simulink model "periodicSwitchTest"  (Simulink 7.9)
settings: Solver=ode45  StartTime=0.0  StopTime=60  MaxStep=0.001  RelTol=1e-3
settings Model: Creator=root  LastModifiedBy=root

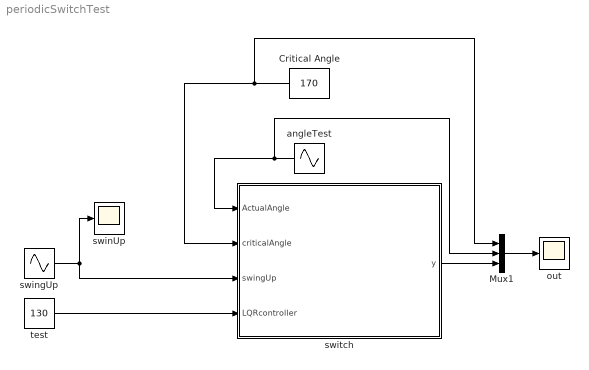
== system periodicSwitchTest ==
  Critical Angle : Constant  Value=170
  Mux1 : Mux  Inputs=3
  angleTest : Sin  Amplitude=20  Bias=160  Frequency=0.1
  out : Scope
      settings: YMin=115  YMax=180
  swinUp : Scope
  swingUp : Sin  Amplitude=2  Bias=120  Frequency=10
  switch : MATLAB Function  TreatAsAtomicUnit=on
  test : Constant  Value=130
  wires:
  swingUp/1 -> swinUp/1, switch/3(swingUp)
  Critical Angle/1 -> switch/2(criticalAngle), Mux1/1
  test/1 -> switch/4(LQRcontroller)
  angleTest/1 -> switch/1(ActualAngle), Mux1/2
  Mux1/1 -> out/1
  switch/1(y) -> Mux1/3

== matlab function switch ==
  data: y output double; ActualAngle input double; criticalAngle input double; swingUp input double; LQRcontroller input double
function y  = fcn(ActualAngle, criticalAngle, swingUp, LQRcontroller)
%function y = fcn(swingUp, LQRcontroller, globalState)
%
if (ActualAngle < criticalAngle)
    y = swingUp;
    %globalStateOut = 0;
else %if (ActualAngle >= criticalAngle || globalState == 1)
    y = LQRcontroller;
    %globalStateOut = 1;
end

end
